simulink model "TRN_current"  (Simulink 6.2)
settings: Solver=ode45  SolverMode=SingleTasking  StartTime=0  StopTime=6  MaxStep=0.1  RelTol=1e-3  AbsTol=1e-3
libraries: simulink x1
(part 1 of 3)
settings Model: LastModifiedBy=mark
settings DataIOCC: LimitDataPoints=off  SaveOutput=off  SaveTime=off  Refine=5
settings OptimizationCC: BooleanDataType=off
settings HardwareCC: TargetUnknown=on
settings RTWCC: TemplateMakefile=grt_unix.tmf
settings GRTTargetCC: ModelReferenceCompliant=off  MatFileLogging=off

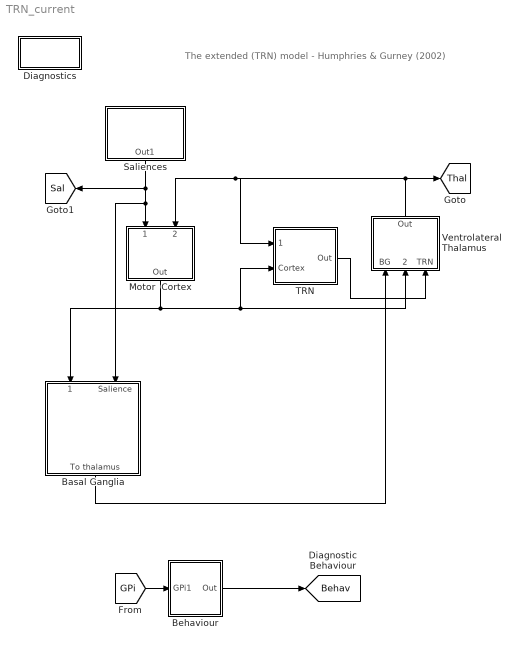
== system TRN_current ==
  note: The extended (TRN) model - Humphries & Gurney (2002)
  Basal Ganglia : Subsystem  Orientation=down  mask(Basal Ganglia){D2=0.2, D1=0.2}
      mask prompts: D2 "D2 base level"; D1 "D1 base level"
  Behaviour : Subsystem  mask(Behaviour expression){on_thresh=0.025, off_thresh=0.1}
      mask prompts: on_thresh "GPi level for behav. on"; off_thresh "GPi level for behav.  off"
  Diagnostics : Subsystem
  Motor  Cortex : Subsystem  Orientation=down  mask(Cortex){W_Thal=1, W_Sal=1, A_rate=25, slope=1, thresh=0}
      mask prompts: W_Thal "Thalamus input weight"; W_Sal "Salience input weight"; A_rate "membrane decay rate"; slope "output slope"; thresh "output thresh"
      mask help: 3 channel striatum - non-recurrent
  Saliences : Subsystem  Orientation=down
  TRN : Subsystem  mask(Thalamic Reticular Nucleus){W_Ctx=1, W_Thal=1, A_rate=25, slope=1, thresh=0}
      mask prompts: W_Ctx "Cortex input weight"; W_Thal "Thalamus input weight"; A_rate "membrane decay rate"; slope "output slope"; thresh "output thresh"
      mask help: 3 channel striatum - non-recurrent
  Ventrolateral Thalamus : Subsystem  Orientation=up  mask(Thalamus){W_TRNwit=-0.1, W_TRNdif=-0.7, W_Ctx=1, W_BG=-1, A_rate=25, slope=1, thresh=0}
      mask prompts: W_TRNwit "Within input weight"; W_TRNdif "Diffuse input weight"; W_Ctx "Cortex input weight"; W_BG "BG input weight"; A_rate "membrane decay rate"; slope "output slope"; thresh "output thresh"
      mask help: 3 channel striatum - non-recurrent
  tag scope: Behav=global, Sal=global, Thal=global
  wires:
  Ventrolateral Thalamus/1(Out) -> [Thal], Motor  Cortex/2(Thalamus), TRN/1(Thalamus)
  [GPi] -> Behaviour/1(GPi1)
  Behaviour/1(Out) -> [Behav]
  Saliences/1(Out1) -> [Sal], Motor  Cortex/1(Salience), Basal Ganglia/2(Salience)
  Motor  Cortex/1(Out) -> Basal Ganglia/1(From cortex), TRN/2(Cortex), Ventrolateral Thalamus/2(Cortex)
  Basal Ganglia/1(To thalamus) -> Ventrolateral Thalamus/1(BG)
  TRN/1(Out) -> Ventrolateral Thalamus/3(TRN)

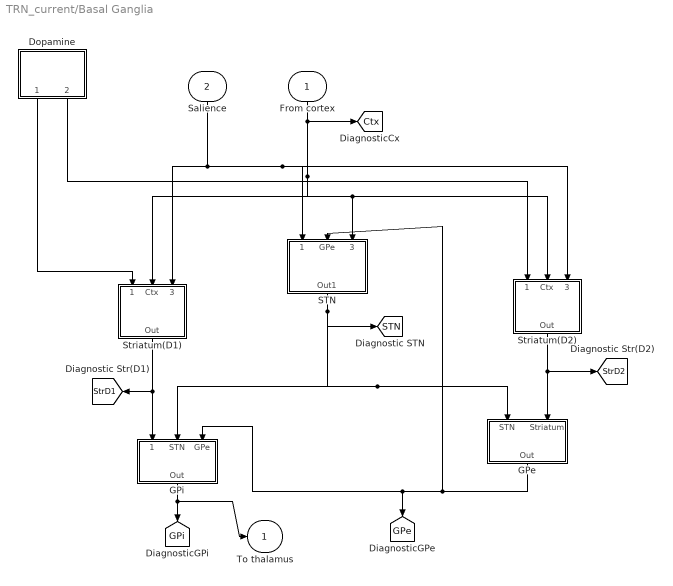
== system TRN_current/Basal Ganglia ==
  From cortex : Inport  Orientation=down  Port=1  SampleTime=0  LatchInput=off
  Salience : Inport  Orientation=down  Port=2  SampleTime=0  LatchInput=off
  Dopamine : Subsystem  Orientation=down
  GPe : Subsystem  Orientation=down  mask(GPe){W_str=-1, W_STN=0.8, A_rate=25, slope=1, thresh=-0.2}
      mask prompts: W_str "weight from Striatum"; W_STN "weight from STN (exc.)"; A_rate "membrane decay rate"; slope "output slope"; thresh "output thresh"
      mask help: 3 channel GPe
  GPi : Subsystem  Orientation=down  mask(GPi){W_str=-1, W_STN=0.8, W_GPe=-0.4, A_rate=25, slope=1, thresh=-0.2}
      mask prompts: W_str "weight from Str"; W_STN "weight from STN"; W_GPe "weight from GPe"; A_rate "membrane decay rate"; slope "output slope"; thresh "output thresh"
      mask help: 3 channel GPe
  STN : Subsystem  Orientation=down
  Striatum(D1) : Subsystem  Orientation=down  mask(Striatum (D1)){W_sal=0.5, W_ctx=0.5, A_rate=25, slope=1, thresh=0.2}
      mask prompts: W_sal "Salience input weight"; W_ctx "Cortex input weight"; A_rate "membrane decay rate"; slope "output slope"; thresh "output thresh"
      mask help: 3 channel striatum - non-recurrent
  Striatum(D2) : Subsystem  Orientation=down  mask(Striatum (D1)){W_sal=0.5, W_ctx=0.5, A_rate=25, slope=1, thresh=0.2}
      mask prompts: W_sal "Salience input weight"; W_ctx "Cortex input weight"; A_rate "membrane decay rate"; slope "output slope"; thresh "output thresh"
      mask help: 3 channel striatum - non-recurrent
  To thalamus : Outport
  tag scope: Ctx=global, GPe=global, GPi=global, STN=global, StrD1=global, StrD2=global
  wires:
  GPe/1(Out) -> STN/2(GPe), GPi/3(GPe), [GPe]
  Striatum(D2)/1(Out) -> GPe/2(Striatum), [StrD2]
  STN/1(Out1) -> [STN], GPe/1(STN), GPi/2(STN)
  Striatum(D1)/1(Out) -> GPi/1(Striatum), [StrD1]
  Dopamine/1(GPi(D1)) -> Striatum(D1)/1(Dopamine)
  Dopamine/2(GPe(D2)) -> Striatum(D2)/1(Dopamine)
  GPi/1(Out) -> [GPi], To thalamus/1
  Salience/1 -> Striatum(D1)/3(Salience), Striatum(D2)/3(Salience), STN/1(saliences)
  From cortex/1 -> [Ctx], Striatum(D1)/2(Ctx), Striatum(D2)/2(Ctx), STN/3(cortex)

== system TRN_current/Behaviour ==
  GPi1 : Inport  Port=1  LatchInput=off
  Constant : Constant
  Relay : Relay  OnSwitchValue=1 - on_thresh  OffSwitchValue=1 - off_thresh
  Sum : Sum  Inputs=+-  SaturateOnIntegerOverflow=on  InputSameDT=on
  Out : Outport  InitialOutput=0
  wires:
  Constant/1 -> Sum/1
  Sum/1 -> Relay/1
  GPi1/1 -> Sum/2
  Relay/1 -> Out/1

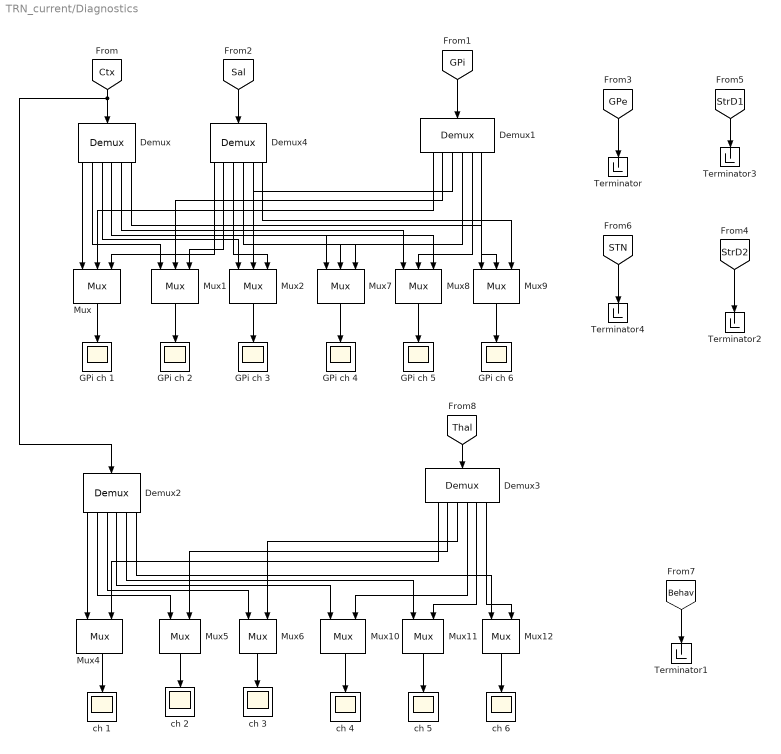
== system TRN_current/Diagnostics ==
  Demux{,1..4} (5 alike) : Demux  Orientation=down  Outputs=6
  GPi ch {1..6} (6 alike) : Scope
      GPi ch 1 settings: Orientation=down  TickLabels=on  YMin=0  YMax=1  SaveName=GPic1_6  DataFormat=Array  MaxDataPoints=7000
      GPi ch 2 settings: Orientation=down  TickLabels=on  YMin=0  YMax=1  SaveName=GPic2_6  DataFormat=Array  MaxDataPoints=7000
      GPi ch 3 settings: Orientation=down  TickLabels=on  YMin=0  YMax=1  SaveName=GPic3_6  DataFormat=Array
      GPi ch 4 settings: Orientation=down  TickLabels=on  YMin=0  YMax=0.75  SaveName=GPic4_6  DataFormat=Array
      GPi ch 5 settings: Orientation=down  TickLabels=on  YMin=0  YMax=0.75  SaveName=GPi3full  DataFormat=Array
      GPi ch 6 settings: Orientation=down  TickLabels=on  YMin=0  YMax=0.75  SaveName=GPi6full6  DataFormat=Array
  Mux{,1..2,7..9} (6 alike) : Mux  Orientation=down  Inputs=3
  Mux{4..6,10..12} (6 alike) : Mux  Orientation=down  Inputs=2
  Terminator{,1..4} (5 alike) : Terminator
      settings: Orientation=down
  ch {1..6} (6 alike) : Scope
      ch 1 settings: Orientation=down  TickLabels=on  YMin=0  YMax=1  SaveName=gpe1  DataFormat=Array
      ch 2 settings: Orientation=down  TickLabels=on  YMin=0  YMax=0.75  SaveName=gpe2  DataFormat=Array
      ch 3 settings: Orientation=down  TickLabels=on  YMin=0  YMax=0.75  SaveName=ch3  DataFormat=Array
      ch 4 settings: Orientation=down  TickLabels=on  YMin=0  YMax=0.75  SaveName=ch4  DataFormat=Array
      ch 5 settings: Orientation=down  TickLabels=on  YMin=0  YMax=0.75  SaveName=ch5  DataFormat=Array
      ch 6 settings: Orientation=down  TickLabels=on  YMin=0  YMax=0.75  SaveName=ch6  DataFormat=Array
  wires:
  [Thal] -> Demux3/1
  Mux/1 -> GPi ch 1/1
  Demux/1 -> Mux/1
  Demux/2 -> Mux1/1
  Mux1/1 -> GPi ch 2/1
  Mux2/1 -> GPi ch 3/1
  Demux/3 -> Mux2/1
  Demux/4 -> Mux7/1
  Demux/5 -> Mux8/1
  Demux/6 -> Mux9/1
  Demux1/3 -> Mux2/2
  [GPi] -> Demux1/1
  Demux1/1 -> Mux/2
  Demux1/2 -> Mux1/2
  Demux1/4 -> Mux7/2
  Demux1/5 -> Mux8/2
  Demux1/6 -> Mux9/2
  Mux7/1 -> GPi ch 4/1
  Mux8/1 -> GPi ch 5/1
  Mux9/1 -> GPi ch 6/1
  [Ctx] -> Demux/1, Demux2/1
  Mux4/1 -> ch 1/1
  Demux2/1 -> Mux4/1
  Demux2/2 -> Mux5/1
  Mux5/1 -> ch 2/1
  Mux6/1 -> ch 3/1
  Demux2/3 -> Mux6/1
  Demux2/4 -> Mux10/1
  Demux2/5 -> Mux11/1
  Demux2/6 -> Mux12/1
  Demux3/3 -> Mux6/2
  Demux3/1 -> Mux4/2
  Demux3/2 -> Mux5/2
  Demux3/4 -> Mux10/2
  Demux3/5 -> Mux11/2
  Demux3/6 -> Mux12/2
  Mux10/1 -> ch 4/1
  Mux11/1 -> ch 5/1
  Mux12/1 -> ch 6/1
  [Sal] -> Demux4/1
  Demux4/1 -> Mux/3
  Demux4/2 -> Mux1/3
  Demux4/3 -> Mux2/3
  Demux4/4 -> Mux7/3
  Demux4/5 -> Mux8/3
  Demux4/6 -> Mux9/3
  [GPe] -> Terminator/1
  [Behav] -> Terminator1/1
  [StrD2] -> Terminator2/1
  [StrD1] -> Terminator3/1
  [STN] -> Terminator4/1

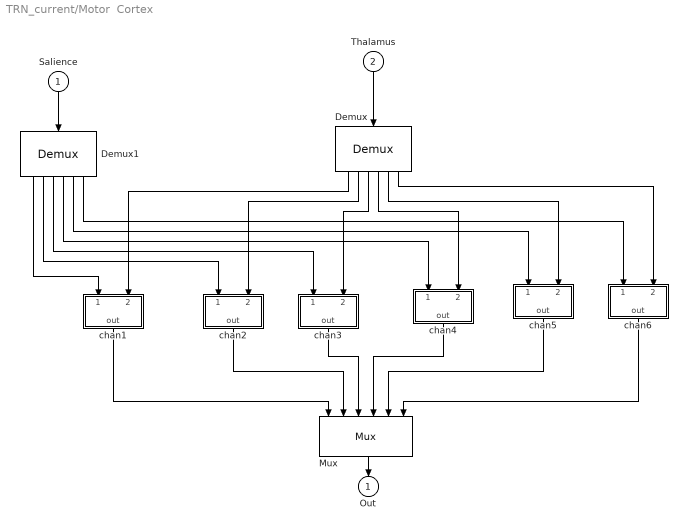
== system TRN_current/Motor  Cortex ==
  Salience : Inport  Orientation=down  Port=1  LatchInput=off
  Thalamus : Inport  Orientation=down  Port=2  LatchInput=off
  Demux : Demux  Orientation=down  Outputs=6
  Demux1 : Demux  Orientation=down  Outputs=6
  Mux : Mux  Orientation=down  Inputs=6
  chan1 : Subsystem  Orientation=down
  chan2 : Subsystem  Orientation=down
  chan3 : Subsystem  Orientation=down
  chan4 : Subsystem  Orientation=down
  chan5 : Subsystem  Orientation=down
  chan6 : Subsystem  Orientation=down
  Out : Outport  Orientation=down  InitialOutput=0
  wires:
  Demux1/1 -> chan1/1(Salience)
  Demux1/2 -> chan2/1(Salience)
  Demux1/3 -> chan3/1(Salience)
  Demux1/4 -> chan4/1(Salience)
  Demux1/5 -> chan5/1(Salience)
  Demux1/6 -> chan6/1(Salience)
  Salience/1 -> Demux1/1
  chan6/1(out) -> Mux/6
  chan5/1(out) -> Mux/5
  chan4/1(out) -> Mux/4
  Demux/6 -> chan6/2(Thalamus)
  Demux/5 -> chan5/2(Thalamus)
  Demux/4 -> chan4/2(Thalamus)
  Demux/3 -> chan3/2(Thalamus)
  Demux/2 -> chan2/2(Thalamus)
  Demux/1 -> chan1/2(Thalamus)
  chan2/1(out) -> Mux/2
  chan3/1(out) -> Mux/3
  Mux/1 -> Out/1
  Thalamus/1 -> Demux/1
  chan1/1(out) -> Mux/1

== system TRN_current/Saliences ==
  Do left : Constant  Orientation=down  Value=0
  Salience (simple) : Subsystem  Orientation=down
  Switch : Switch  Orientation=down  Threshold=0.5  SaturateOnIntegerOverflow=on  InputSameDT=on
  step pairs : Subsystem  Orientation=down
  Out1 : Outport  Orientation=down  InitialOutput=0
  wires:
  Switch/1 -> Out1/1
  Salience (simple)/1(out) -> Switch/3
  step pairs/1(out) -> Switch/1
  Do left/1 -> Switch/2

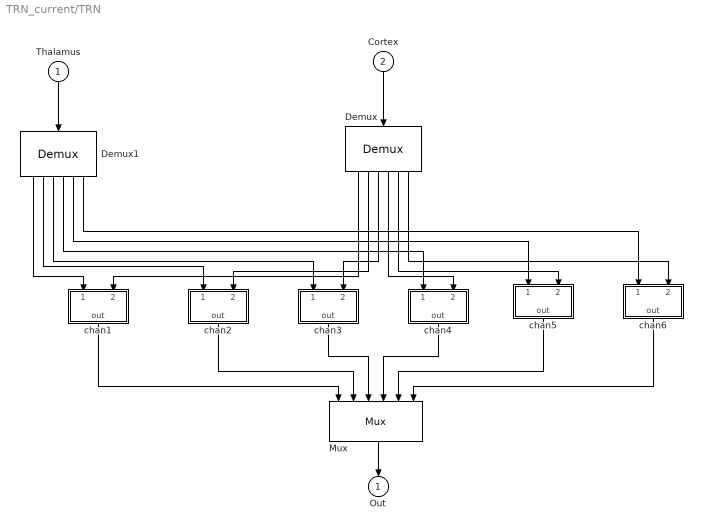
== system TRN_current/TRN ==
  Thalamus : Inport  Orientation=down  Port=1  LatchInput=off
  Cortex : Inport  Orientation=down  Port=2  LatchInput=off
  Demux : Demux  Orientation=down  Outputs=6
  Demux1 : Demux  Orientation=down  Outputs=6
  Mux : Mux  Orientation=down  Inputs=6
  chan1 : Subsystem  Orientation=down
  chan2 : Subsystem  Orientation=down
  chan3 : Subsystem  Orientation=down
  chan4 : Subsystem  Orientation=down
  chan5 : Subsystem  Orientation=down
  chan6 : Subsystem  Orientation=down
  Out : Outport  Orientation=down  InitialOutput=0
  wires:
  Demux/1 -> chan1/2(Cortex)
  Demux1/1 -> chan1/1(Thalamus)
  Mux/1 -> Out/1
  chan1/1(out) -> Mux/1
  chan3/1(out) -> Mux/3
  chan2/1(out) -> Mux/2
  chan4/1(out) -> Mux/4
  chan5/1(out) -> Mux/5
  chan6/1(out) -> Mux/6
  Cortex/1 -> Demux/1
  Thalamus/1 -> Demux1/1
  Demux1/2 -> chan2/1(Thalamus)
  Demux1/3 -> chan3/1(Thalamus)
  Demux1/4 -> chan4/1(Thalamus)
  Demux1/5 -> chan5/1(Thalamus)
  Demux1/6 -> chan6/1(Thalamus)
  Demux/2 -> chan2/2(Cortex)
  Demux/3 -> chan3/2(Cortex)
  Demux/4 -> chan4/2(Cortex)
  Demux/5 -> chan5/2(Cortex)
  Demux/6 -> chan6/2(Cortex)

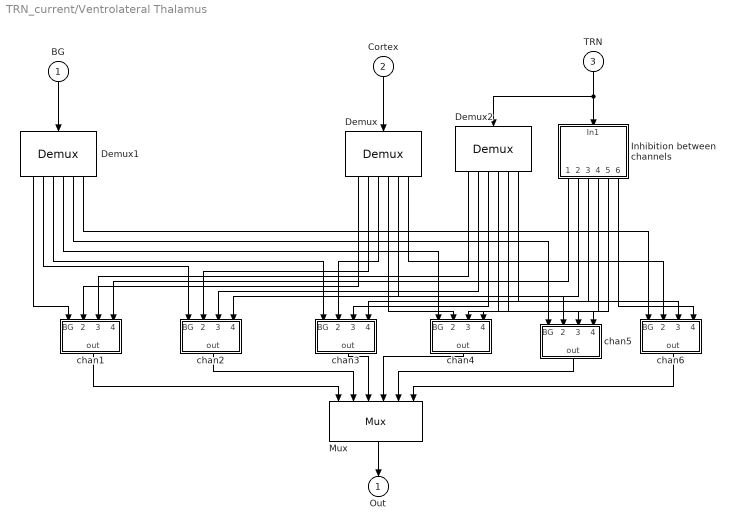
== system TRN_current/Ventrolateral Thalamus ==
  BG : Inport  Orientation=down  Port=1  LatchInput=off
  Cortex : Inport  Orientation=down  Port=2  LatchInput=off
  TRN : Inport  Orientation=down  Port=3  LatchInput=off
  Demux : Demux  Orientation=down  Outputs=6
  Demux1 : Demux  Orientation=down  Outputs=6
  Demux2 : Demux  Orientation=down  Outputs=6
  Inhibition between channels : Subsystem  Orientation=down
  Mux : Mux  Orientation=down  Inputs=6
  chan1 : Subsystem  Orientation=down
  chan2 : Subsystem  Orientation=down
  chan3 : Subsystem  Orientation=down
  chan4 : Subsystem  Orientation=down
  chan5 : Subsystem  Orientation=down
  chan6 : Subsystem  Orientation=down
  Out : Outport  Orientation=down  InitialOutput=0
  wires:
  Mux/1 -> Out/1
  chan1/1(out) -> Mux/1
  chan3/1(out) -> Mux/3
  chan2/1(out) -> Mux/2
  chan4/1(out) -> Mux/4
  chan5/1(out) -> Mux/5
  chan6/1(out) -> Mux/6
  BG/1 -> Demux1/1
  Demux1/2 -> chan2/1(BG)
  Demux1/3 -> chan3/1(BG)
  Demux1/4 -> chan4/1(BG)
  Demux1/5 -> chan5/1(BG)
  Cortex/1 -> Demux/1
  Demux1/6 -> chan6/1(BG)
  Demux1/1 -> chan1/1(BG)
  TRN/1 -> Inhibition between channels/1(In1), Demux2/1
  Demux2/1 -> chan1/3(TRN)
  Inhibition between channels/1(Out1) -> chan1/4(TRN1)
  Demux2/2 -> chan2/3(TRN)
  Demux2/3 -> chan3/3(TRN)
  Demux2/4 -> chan4/3(TRN)
  Demux2/5 -> chan5/3(TRN)
  Demux2/6 -> chan6/3(TRN)
  Inhibition between channels/2(Out2) -> chan2/4(TRN1)
  Inhibition between channels/3(Out3) -> chan3/4(TRN1)
  Inhibition between channels/4(Out4) -> chan4/4(TRN1)
  Inhibition between channels/5(Out5) -> chan5/4(TRN1)
  Inhibition between channels/6(Out6) -> chan6/4(TRN1)
  Demux/2 -> chan2/2(Cortex)
  Demux/3 -> chan3/2(Cortex)
  Demux/4 -> chan4/2(Cortex)
  Demux/5 -> chan5/2(Cortex)
  Demux/6 -> chan6/2(Cortex)
  Demux/1 -> chan1/2(Cortex)

== system TRN_current/Basal Ganglia/Dopamine ==
  D1 base level : Constant  Value=D1
  D2 base level : Constant  Orientation=left  Value=D2
  Mux : Mux  Orientation=down  Inputs=6
  Mux1 : Mux  Orientation=down  Inputs=6
  GPi(D1) : Outport  Orientation=down  InitialOutput=0
  GPe(D2) : Outport  Orientation=down  Port=2  InitialOutput=0
  wires:
  Mux1/1 -> GPe(D2)/1
  D2 base level/1 -> Mux1/6, Mux1/5, Mux1/4, Mux1/3, Mux1/2, Mux1/1
  Mux/1 -> GPi(D1)/1
  D1 base level/1 -> Mux/6, Mux/5, Mux/4, Mux/3, Mux/2, Mux/1

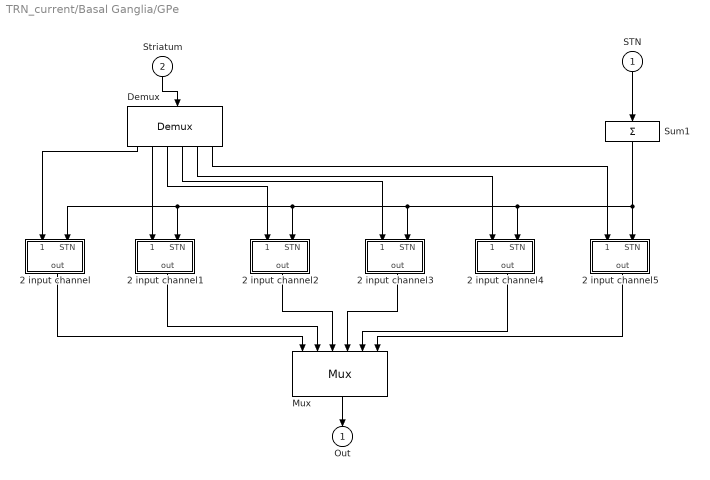
== system TRN_current/Basal Ganglia/GPe ==
  STN : Inport  Orientation=down  Port=1  LatchInput=off
  Striatum : Inport  Orientation=down  Port=2  LatchInput=off
  2 input channel : Subsystem  Orientation=down
  2 input channel1 : Subsystem  Orientation=down
  2 input channel2 : Subsystem  Orientation=down
  2 input channel3 : Subsystem  Orientation=down
  2 input channel4 : Subsystem  Orientation=down
  2 input channel5 : Subsystem  Orientation=down
  Demux : Demux  Orientation=down  Outputs=6
  Mux : Mux  Orientation=down  Inputs=6
  Sum1 : Sum  Orientation=down  Inputs=+  SaturateOnIntegerOverflow=on  InputSameDT=on
  Out : Outport  Orientation=down  InitialOutput=0
  wires:
  Sum1/1 -> 2 input channel5/2(STN), 2 input channel/2(STN), 2 input channel1/2(STN), 2 input channel2/2(STN), 2 input channel3/2(STN), 2 input channel4/2(STN)
  Demux/1 -> 2 input channel/1(Striatum)
  STN/1 -> Sum1/1
  2 input channel/1(out) -> Mux/1
  2 input channel1/1(out) -> Mux/2
  2 input channel2/1(out) -> Mux/3
  Mux/1 -> Out/1
  Striatum/1 -> Demux/1
  Demux/2 -> 2 input channel1/1(Striatum)
  Demux/3 -> 2 input channel2/1(Striatum)
  Demux/4 -> 2 input channel3/1(Striatum)
  Demux/5 -> 2 input channel4/1(Striatum)
  Demux/6 -> 2 input channel5/1(Striatum)
  2 input channel3/1(out) -> Mux/4
  2 input channel4/1(out) -> Mux/5
  2 input channel5/1(out) -> Mux/6

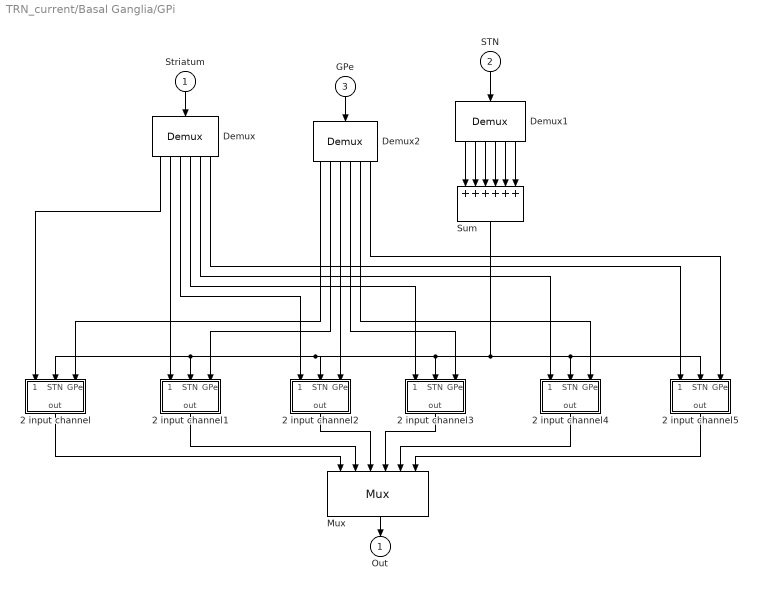
== system TRN_current/Basal Ganglia/GPi ==
  Striatum : Inport  Orientation=down  Port=1  LatchInput=off
  STN : Inport  Orientation=down  Port=2  LatchInput=off
  GPe : Inport  Orientation=down  Port=3  LatchInput=off
  2 input channel : Subsystem  Orientation=down
  2 input channel1 : Subsystem  Orientation=down
  2 input channel2 : Subsystem  Orientation=down
  2 input channel3 : Subsystem  Orientation=down
  2 input channel4 : Subsystem  Orientation=down
  2 input channel5 : Subsystem  Orientation=down
  Demux : Demux  Orientation=down  Outputs=6
  Demux1 : Demux  Orientation=down  Outputs=6
  Demux2 : Demux  Orientation=down  Outputs=6
  Mux : Mux  Orientation=down  Inputs=6
  Sum : Sum  Orientation=down  Inputs=++++++  SaturateOnIntegerOverflow=on  InputSameDT=on
  Out : Outport  Orientation=down  InitialOutput=0
  wires:
  Mux/1 -> Out/1
  2 input channel2/1(out) -> Mux/3
  2 input channel1/1(out) -> Mux/2
  2 input channel/1(out) -> Mux/1
  GPe/1 -> Demux2/1
  Demux2/1 -> 2 input channel/3(GPe)
  Demux2/2 -> 2 input channel1/3(GPe)
  Demux2/3 -> 2 input channel2/3(GPe)
  Demux/2 -> 2 input channel1/1(Striatum)
  Demux/1 -> 2 input channel/1(Striatum)
  Striatum/1 -> Demux/1
  Demux/3 -> 2 input channel2/1(Striatum)
  Demux/4 -> 2 input channel3/1(Striatum)
  Demux/5 -> 2 input channel4/1(Striatum)
  Demux/6 -> 2 input channel5/1(Striatum)
  Demux2/4 -> 2 input channel3/3(GPe)
  Demux2/5 -> 2 input channel4/3(GPe)
  Demux1/1 -> Sum/1
  Demux1/2 -> Sum/2
  Demux1/3 -> Sum/3
  Demux1/4 -> Sum/4
  Demux1/5 -> Sum/5
  Demux1/6 -> Sum/6
  STN/1 -> Demux1/1
  Sum/1 -> 2 input channel/2(STN), 2 input channel1/2(STN), 2 input channel2/2(STN), 2 input channel3/2(STN), 2 input channel4/2(STN), 2 input channel5/2(STN)
  Demux2/6 -> 2 input channel5/3(GPe)
  2 input channel3/1(out) -> Mux/4
  2 input channel4/1(out) -> Mux/5
  2 input channel5/1(out) -> Mux/6

== system TRN_current/Basal Ganglia/STN ==
  saliences : Inport  Orientation=down  Port=1  LatchInput=off
  GPe : Inport  Orientation=down  Port=2  LatchInput=off
  cortex : Inport  Orientation=down  Port=3  LatchInput=off
  STN discrete model : Subsystem  Orientation=down  mask(STN){W_sal=0.5, W_Ctx=0.5, W_GPe=-1, A_rate=25, slope=1, thresh=-0.25}
      mask prompts: W_sal "weight from salience"; W_Ctx "weight from Cortex"; W_GPe "weight from GPe(inhib.)"; A_rate "membrane decay rate"; slope "output slope"; thresh "output thresh"
      mask help: 3 channel GPe
  Out1 : Outport  Orientation=down  InitialOutput=0
  wires:
  GPe/1 -> STN discrete model/2(GPe)
  saliences/1 -> STN discrete model/1(Saliences)
  STN discrete model/1(Out) -> Out1/1
  cortex/1 -> STN discrete model/3(Cortex)

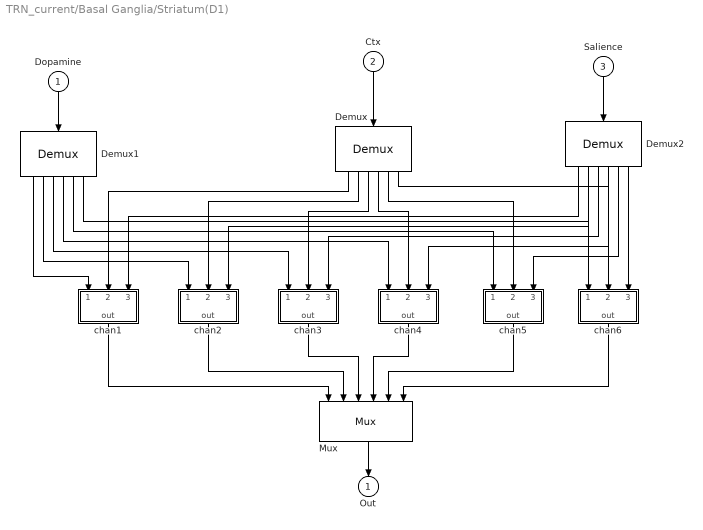
== system TRN_current/Basal Ganglia/Striatum(D1) ==
  Dopamine : Inport  Orientation=down  Port=1  LatchInput=off
  Ctx : Inport  Orientation=down  Port=2  LatchInput=off
  Salience : Inport  Orientation=down  Port=3  LatchInput=off
  Demux : Demux  Orientation=down  Outputs=6
  Demux1 : Demux  Orientation=down  Outputs=6
  Demux2 : Demux  Orientation=down  Outputs=6
  Mux : Mux  Orientation=down  Inputs=6
  chan1 : Subsystem  Orientation=down
  chan2 : Subsystem  Orientation=down
  chan3 : Subsystem  Orientation=down
  chan4 : Subsystem  Orientation=down
  chan5 : Subsystem  Orientation=down
  chan6 : Subsystem  Orientation=down
  Out : Outport  Orientation=down  InitialOutput=0
  wires:
  Ctx/1 -> Demux/1
  Mux/1 -> Out/1
  chan1/1(out) -> Mux/1
  chan3/1(out) -> Mux/3
  chan2/1(out) -> Mux/2
  Demux/2 -> chan2/2(cortex)
  Demux/3 -> chan3/2(cortex)
  Demux/4 -> chan4/2(cortex)
  Demux/5 -> chan5/2(cortex)
  Demux/6 -> chan6/2(cortex)
  chan4/1(out) -> Mux/4
  chan5/1(out) -> Mux/5
  chan6/1(out) -> Mux/6
  Dopamine/1 -> Demux1/1
  Demux1/6 -> chan6/1(dopamine)
  Demux1/5 -> chan5/1(dopamine)
  Demux1/4 -> chan4/1(dopamine)
  Demux1/3 -> chan3/1(dopamine)
  Demux1/2 -> chan2/1(dopamine)
  Demux1/1 -> chan1/1(dopamine)
  Salience/1 -> Demux2/1
  Demux2/2 -> chan2/3(salience)
  Demux2/3 -> chan3/3(salience)
  Demux2/4 -> chan4/3(salience)
  Demux2/5 -> chan5/3(salience)
  Demux2/6 -> chan6/3(salience)
  Demux/1 -> chan1/2(cortex)
  Demux2/1 -> chan1/3(salience)

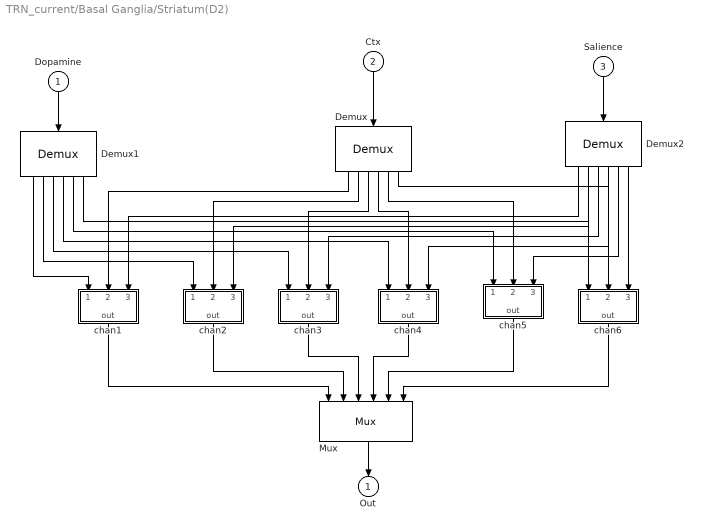
== system TRN_current/Basal Ganglia/Striatum(D2) ==
  Dopamine : Inport  Orientation=down  Port=1  LatchInput=off
  Ctx : Inport  Orientation=down  Port=2  LatchInput=off
  Salience : Inport  Orientation=down  Port=3  LatchInput=off
  Demux : Demux  Orientation=down  Outputs=6
  Demux1 : Demux  Orientation=down  Outputs=6
  Demux2 : Demux  Orientation=down  Outputs=6
  Mux : Mux  Orientation=down  Inputs=6
  chan1 : Subsystem  Orientation=down
  chan2 : Subsystem  Orientation=down
  chan3 : Subsystem  Orientation=down
  chan4 : Subsystem  Orientation=down
  chan5 : Subsystem  Orientation=down
  chan6 : Subsystem  Orientation=down
  Out : Outport  Orientation=down  InitialOutput=0
  wires:
  Demux2/1 -> chan1/3(salience)
  Demux/1 -> chan1/2(cortex)
  Demux2/6 -> chan6/3(salience)
  Demux2/5 -> chan5/3(salience)
  Demux2/4 -> chan4/3(salience)
  Demux2/3 -> chan3/3(salience)
  Demux2/2 -> chan2/3(salience)
  Salience/1 -> Demux2/1
  Demux1/1 -> chan1/1(dopamine)
  Demux1/2 -> chan2/1(dopamine)
  Demux1/3 -> chan3/1(dopamine)
  Demux1/4 -> chan4/1(dopamine)
  Demux1/5 -> chan5/1(dopamine)
  Demux1/6 -> chan6/1(dopamine)
  Dopamine/1 -> Demux1/1
  chan6/1(out) -> Mux/6
  chan5/1(out) -> Mux/5
  chan4/1(out) -> Mux/4
  Demux/6 -> chan6/2(cortex)
  Demux/5 -> chan5/2(cortex)
  Demux/4 -> chan4/2(cortex)
  Demux/3 -> chan3/2(cortex)
  Demux/2 -> chan2/2(cortex)
  chan2/1(out) -> Mux/2
  chan3/1(out) -> Mux/3
  chan1/1(out) -> Mux/1
  Mux/1 -> Out/1
  Ctx/1 -> Demux/1

== system TRN_current/Motor  Cortex/chan1 ==
  Salience : Inport  Orientation=down  Port=1  PortDimensions=1  LatchInput=off
  Thalamus : Inport  Orientation=down  Port=2  LatchInput=off
  Sum : Sum  Orientation=down  SaturateOnIntegerOverflow=on  InputSameDT=on
  leaky integration : Subsystem  Orientation=down
  piecewise lin.1 : S-Function  Orientation=down  FunctionName=Mpieclin  Parameters=slope,thresh
  weight : Gain  Orientation=down  Gain=W_Thal  SaturateOnIntegerOverflow=on
  weight1 : Gain  Orientation=down  Gain=W_Sal  SaturateOnIntegerOverflow=on
  out : Outport  Orientation=down  InitialOutput=0
  wires:
  Thalamus/1 -> weight/1
  Salience/1 -> weight1/1
  weight/1 -> Sum/2
  weight1/1 -> Sum/1
  piecewise lin.1/1 -> out/1
  Sum/1 -> leaky integration/1(Inport)
  leaky integration/1(Outport) -> piecewise lin.1/1

== system TRN_current/Motor  Cortex/chan2 ==
  Salience : Inport  Orientation=down  Port=1  PortDimensions=1  LatchInput=off
  Thalamus : Inport  Orientation=down  Port=2  LatchInput=off
  Sum : Sum  Orientation=down  SaturateOnIntegerOverflow=on  InputSameDT=on
  leaky integration : Subsystem  Orientation=down
  piecewise lin.1 : S-Function  Orientation=down  FunctionName=Mpieclin  Parameters=slope,thresh
  weight : Gain  Orientation=down  Gain=W_Thal  SaturateOnIntegerOverflow=on
  weight1 : Gain  Orientation=down  Gain=W_Sal  SaturateOnIntegerOverflow=on
  out : Outport  Orientation=down  InitialOutput=0
  wires:
  leaky integration/1(Outport) -> piecewise lin.1/1
  Sum/1 -> leaky integration/1(Inport)
  piecewise lin.1/1 -> out/1
  weight1/1 -> Sum/1
  weight/1 -> Sum/2
  Salience/1 -> weight1/1
  Thalamus/1 -> weight/1

== system TRN_current/Motor  Cortex/chan3 ==
  Salience : Inport  Orientation=down  Port=1  PortDimensions=1  LatchInput=off
  Thalamus : Inport  Orientation=down  Port=2  LatchInput=off
  Sum : Sum  Orientation=down  SaturateOnIntegerOverflow=on  InputSameDT=on
  leaky integration : Subsystem  Orientation=down
  piecewise lin.1 : S-Function  Orientation=down  FunctionName=Mpieclin  Parameters=slope,thresh
  weight : Gain  Orientation=down  Gain=W_Thal  SaturateOnIntegerOverflow=on
  weight1 : Gain  Orientation=down  Gain=W_Sal  SaturateOnIntegerOverflow=on
  out : Outport  Orientation=down  InitialOutput=0
  wires:
  Thalamus/1 -> weight/1
  Salience/1 -> weight1/1
  weight/1 -> Sum/2
  weight1/1 -> Sum/1
  piecewise lin.1/1 -> out/1
  Sum/1 -> leaky integration/1(Inport)
  leaky integration/1(Outport) -> piecewise lin.1/1

== system TRN_current/Motor  Cortex/chan4 ==
  Salience : Inport  Orientation=down  Port=1  PortDimensions=1  LatchInput=off
  Thalamus : Inport  Orientation=down  Port=2  LatchInput=off
  Sum : Sum  Orientation=down  SaturateOnIntegerOverflow=on  InputSameDT=on
  leaky integration : Subsystem  Orientation=down
  piecewise lin.1 : S-Function  Orientation=down  FunctionName=Mpieclin  Parameters=slope,thresh
  weight : Gain  Orientation=down  Gain=W_Thal  SaturateOnIntegerOverflow=on
  weight1 : Gain  Orientation=down  Gain=W_Sal  SaturateOnIntegerOverflow=on
  out : Outport  Orientation=down  InitialOutput=0
  wires:
  leaky integration/1(Outport) -> piecewise lin.1/1
  Sum/1 -> leaky integration/1(Inport)
  piecewise lin.1/1 -> out/1
  weight1/1 -> Sum/1
  weight/1 -> Sum/2
  Salience/1 -> weight1/1
  Thalamus/1 -> weight/1

== system TRN_current/Motor  Cortex/chan5 ==
  Salience : Inport  Orientation=down  Port=1  PortDimensions=1  LatchInput=off
  Thalamus : Inport  Orientation=down  Port=2  LatchInput=off
  Sum : Sum  Orientation=down  SaturateOnIntegerOverflow=on  InputSameDT=on
  leaky integration : Subsystem  Orientation=down
  piecewise lin.1 : S-Function  Orientation=down  FunctionName=Mpieclin  Parameters=slope,thresh
  weight : Gain  Orientation=down  Gain=W_Thal  SaturateOnIntegerOverflow=on
  weight1 : Gain  Orientation=down  Gain=W_Sal  SaturateOnIntegerOverflow=on
  out : Outport  Orientation=down  InitialOutput=0
  wires:
  Thalamus/1 -> weight/1
  Salience/1 -> weight1/1
  weight/1 -> Sum/2
  weight1/1 -> Sum/1
  piecewise lin.1/1 -> out/1
  Sum/1 -> leaky integration/1(Inport)
  leaky integration/1(Outport) -> piecewise lin.1/1

== system TRN_current/Motor  Cortex/chan6 ==
  Salience : Inport  Orientation=down  Port=1  PortDimensions=1  LatchInput=off
  Thalamus : Inport  Orientation=down  Port=2  LatchInput=off
  Sum : Sum  Orientation=down  SaturateOnIntegerOverflow=on  InputSameDT=on
  leaky integration : Subsystem  Orientation=down
  piecewise lin.1 : S-Function  Orientation=down  FunctionName=Mpieclin  Parameters=slope,thresh
  weight : Gain  Orientation=down  Gain=W_Thal  SaturateOnIntegerOverflow=on
  weight1 : Gain  Orientation=down  Gain=W_Sal  SaturateOnIntegerOverflow=on
  out : Outport  Orientation=down  InitialOutput=0
  wires:
  leaky integration/1(Outport) -> piecewise lin.1/1
  Sum/1 -> leaky integration/1(Inport)
  piecewise lin.1/1 -> out/1
  weight1/1 -> Sum/1
  weight/1 -> Sum/2
  Salience/1 -> weight1/1
  Thalamus/1 -> weight/1

== system TRN_current/Saliences/Salience (simple) ==
  Saliences : DiscretePulseGenerator  Orientation=down  PulseType=Time based  Amplitude=[0.4 0.42 0.0 0.0 0.0 0.0]  Period=10  PulseWidth=[90 90 90 90 90 90]  PhaseDelay=[1 1 4 3 3 4]
  Sum : Sum  Orientation=down  SaturateOnIntegerOverflow=on  InputSameDT=on
  Transients : DiscretePulseGenerator  Orientation=down  PulseType=Time based  Amplitude=[0.2 0.0 0 0 0 0]  Period=10  PulseWidth=[10 30 10 10 10 10]  PhaseDelay=[4 5 10 10 10 10]
  out : Outport  Orientation=down  InitialOutput=0
  wires:
  ? -> Sum/2
  Sum/1 -> out/1
  Saliences/1 -> Sum/1

== system TRN_current/Saliences/step pairs ==
  Constant : Constant  Orientation=down  Value=[0 0 0 0 ]
  Constant1 : Constant  Orientation=down  Value=0.4
  Mux : Mux  Orientation=down  Inputs=3
  Repeating Sequence : simulink/Sources/Repeating Sequence  Orientation=down  rep_seq_t=[0 0.5 1.0 1.5 2.0 2.5 3.0 3.5 4 4.5 5]  rep_seq_y=[0 0.1 0.2 0.3 0.4 0.5 0.6 0.7 0.8 0.9 1]
  Scope : Scope
      settings: TickLabels=on  DataFormat=Array
  Zero-Order Hold : ZeroOrderHold  Orientation=down  SampleTime=0.5
  out : Outport  Orientation=down  InitialOutput=0
  wires:
  Mux/1 -> out/1, Scope/1
  Constant/1 -> Mux/3
  Repeating Sequence/1 -> Zero-Order Hold/1
  Zero-Order Hold/1 -> Mux/2
  Constant1/1 -> Mux/1

== system TRN_current/TRN/chan1 ==
  Thalamus : Inport  Orientation=down  Port=1  LatchInput=off
  Cortex : Inport  Orientation=down  Port=2  LatchInput=off
  Sum : Sum  Orientation=down  SaturateOnIntegerOverflow=on  InputSameDT=on
  leaky integration : Subsystem  Orientation=down
  piecewise lin. : S-Function  Orientation=down  FunctionName=Mpieclin  Parameters=slope,thresh
  weight : Gain  Orientation=down  Gain=W_Ctx  SaturateOnIntegerOverflow=on
  weight1 : Gain  Orientation=down  Gain=W_Thal  SaturateOnIntegerOverflow=on
  out : Outport  Orientation=down  InitialOutput=0
  wires:
  Cortex/1 -> weight/1
  leaky integration/1(Outport) -> piecewise lin./1
  weight1/1 -> Sum/1
  weight/1 -> Sum/2
  Sum/1 -> leaky integration/1(Inport)
  piecewise lin./1 -> out/1
  Thalamus/1 -> weight1/1

== system TRN_current/TRN/chan2 ==
  Thalamus : Inport  Orientation=down  Port=1  LatchInput=off
  Cortex : Inport  Orientation=down  Port=2  LatchInput=off
  Sum : Sum  Orientation=down  SaturateOnIntegerOverflow=on  InputSameDT=on
  leaky integration : Subsystem  Orientation=down
  piecewise lin. : S-Function  Orientation=down  FunctionName=Mpieclin  Parameters=slope,thresh
  weight : Gain  Orientation=down  Gain=W_Ctx  SaturateOnIntegerOverflow=on
  weight1 : Gain  Orientation=down  Gain=W_Thal  SaturateOnIntegerOverflow=on
  out : Outport  Orientation=down  InitialOutput=0
  wires:
  Thalamus/1 -> weight1/1
  piecewise lin./1 -> out/1
  Sum/1 -> leaky integration/1(Inport)
  weight/1 -> Sum/2
  weight1/1 -> Sum/1
  leaky integration/1(Outport) -> piecewise lin./1
  Cortex/1 -> weight/1

== system TRN_current/TRN/chan3 ==
  Thalamus : Inport  Orientation=down  Port=1  LatchInput=off
  Cortex : Inport  Orientation=down  Port=2  LatchInput=off
  Sum : Sum  Orientation=down  SaturateOnIntegerOverflow=on  InputSameDT=on
  leaky integration : Subsystem  Orientation=down
  piecewise lin. : S-Function  Orientation=down  FunctionName=Mpieclin  Parameters=slope,thresh
  weight : Gain  Orientation=down  Gain=W_Ctx  SaturateOnIntegerOverflow=on
  weight1 : Gain  Orientation=down  Gain=W_Thal  SaturateOnIntegerOverflow=on
  out : Outport  Orientation=down  InitialOutput=0
  wires:
  Cortex/1 -> weight/1
  leaky integration/1(Outport) -> piecewise lin./1
  weight1/1 -> Sum/1
  weight/1 -> Sum/2
  Sum/1 -> leaky integration/1(Inport)
  piecewise lin./1 -> out/1
  Thalamus/1 -> weight1/1

== system TRN_current/TRN/chan4 ==
  Thalamus : Inport  Orientation=down  Port=1  LatchInput=off
  Cortex : Inport  Orientation=down  Port=2  LatchInput=off
  Sum : Sum  Orientation=down  SaturateOnIntegerOverflow=on  InputSameDT=on
  leaky integration : Subsystem  Orientation=down
  piecewise lin. : S-Function  Orientation=down  FunctionName=Mpieclin  Parameters=slope,thresh
  weight : Gain  Orientation=down  Gain=W_Ctx  SaturateOnIntegerOverflow=on
  weight1 : Gain  Orientation=down  Gain=W_Thal  SaturateOnIntegerOverflow=on
  out : Outport  Orientation=down  InitialOutput=0
  wires:
  Thalamus/1 -> weight1/1
  piecewise lin./1 -> out/1
  Sum/1 -> leaky integration/1(Inport)
  weight/1 -> Sum/2
  weight1/1 -> Sum/1
  leaky integration/1(Outport) -> piecewise lin./1
  Cortex/1 -> weight/1

== system TRN_current/TRN/chan5 ==
  Thalamus : Inport  Orientation=down  Port=1  LatchInput=off
  Cortex : Inport  Orientation=down  Port=2  LatchInput=off
  Sum : Sum  Orientation=down  SaturateOnIntegerOverflow=on  InputSameDT=on
  leaky integration : Subsystem  Orientation=down
  piecewise lin. : S-Function  Orientation=down  FunctionName=Mpieclin  Parameters=slope,thresh
  weight : Gain  Orientation=down  Gain=W_Ctx  SaturateOnIntegerOverflow=on
  weight1 : Gain  Orientation=down  Gain=W_Thal  SaturateOnIntegerOverflow=on
  out : Outport  Orientation=down  InitialOutput=0
  wires:
  Cortex/1 -> weight/1
  leaky integration/1(Outport) -> piecewise lin./1
  weight1/1 -> Sum/1
  weight/1 -> Sum/2
  Sum/1 -> leaky integration/1(Inport)
  piecewise lin./1 -> out/1
  Thalamus/1 -> weight1/1

== system TRN_current/TRN/chan6 ==
  Thalamus : Inport  Orientation=down  Port=1  LatchInput=off
  Cortex : Inport  Orientation=down  Port=2  LatchInput=off
  Sum : Sum  Orientation=down  SaturateOnIntegerOverflow=on  InputSameDT=on
  leaky integration : Subsystem  Orientation=down
  piecewise lin. : S-Function  Orientation=down  FunctionName=Mpieclin  Parameters=slope,thresh
  weight : Gain  Orientation=down  Gain=W_Ctx  SaturateOnIntegerOverflow=on
  weight1 : Gain  Orientation=down  Gain=W_Thal  SaturateOnIntegerOverflow=on
  out : Outport  Orientation=down  InitialOutput=0
  wires:
  Thalamus/1 -> weight1/1
  piecewise lin./1 -> out/1
  Sum/1 -> leaky integration/1(Inport)
  weight/1 -> Sum/2
  weight1/1 -> Sum/1
  leaky integration/1(Outport) -> piecewise lin./1
  Cortex/1 -> weight/1

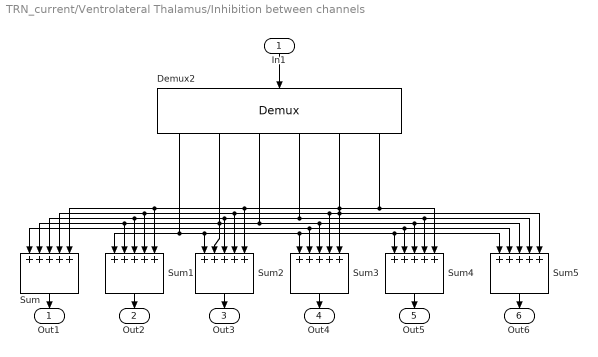
== system TRN_current/Ventrolateral Thalamus/Inhibition between channels ==
  In1 : Inport  Orientation=down  Port=1  LatchInput=off
  Demux2 : Demux  Orientation=down  Outputs=6
  Sum{,1..5} (6 alike) : Sum  Orientation=down  Inputs=+++++  SaturateOnIntegerOverflow=on  InputSameDT=on
  Out1 : Outport  Orientation=down  InitialOutput=0
  Out2 : Outport  Orientation=down  Port=2  InitialOutput=0
  Out3 : Outport  Orientation=down  Port=3  InitialOutput=0
  Out4 : Outport  Orientation=down  Port=4  InitialOutput=0
  Out5 : Outport  Orientation=down  Port=5  InitialOutput=0
  Out6 : Outport  Orientation=down  Port=6  InitialOutput=0
  wires:
  In1/1 -> Demux2/1
  Sum/1 -> Out1/1
  Demux2/2 -> Sum/1, Sum2/2, Sum3/2, Sum4/2, Sum5/2
  Demux2/1 -> Sum1/1, Sum2/1, Sum3/1, Sum4/1, Sum5/1
  Demux2/3 -> Sum/2, Sum1/2, Sum3/3, Sum4/3, Sum5/3
  Demux2/4 -> Sum/3, Sum1/3, Sum2/3, Sum4/4, Sum5/4
  Demux2/5 -> Sum/4, Sum1/4, Sum2/4, Sum3/4, Sum5/5
  Demux2/6 -> Sum/5, Sum1/5, Sum2/5, Sum3/5, Sum4/5
  Sum1/1 -> Out2/1
  Sum2/1 -> Out3/1
  Sum3/1 -> Out4/1
  Sum4/1 -> Out5/1
  Sum5/1 -> Out6/1

== system TRN_current/Ventrolateral Thalamus/chan1 ==
  BG : Inport  Orientation=down  Port=1  LatchInput=off
  Cortex : Inport  Orientation=down  Port=2  LatchInput=off
  TRN : Inport  Orientation=down  Port=3  LatchInput=off
  TRN1 : Inport  Orientation=down  Port=4  LatchInput=off
  Sum : Sum  Orientation=down  Inputs=++++  SaturateOnIntegerOverflow=on  InputSameDT=on
  leaky integration : Subsystem  Orientation=down
  piecewise lin. : S-Function  Orientation=down  FunctionName=Mpieclin  Parameters=slope,thresh
  weight : Gain  Orientation=down  Gain=W_Ctx  SaturateOnIntegerOverflow=on
  weight1 : Gain  Orientation=down  Gain=W_BG  SaturateOnIntegerOverflow=on
  weight2 : Gain  Orientation=down  Gain=W_TRNwit  SaturateOnIntegerOverflow=on
  weight3 : Gain  Orientation=down  Gain=W_TRNdif  SaturateOnIntegerOverflow=on
  out : Outport  Orientation=down  InitialOutput=0
  wires:
  leaky integration/1(Outport) -> piecewise lin./1
  weight1/1 -> Sum/1
  weight/1 -> Sum/2
  BG/1 -> weight1/1
  Cortex/1 -> weight/1
  weight2/1 -> Sum/3
  TRN/1 -> weight2/1
  TRN1/1 -> weight3/1
  weight3/1 -> Sum/4
  Sum/1 -> leaky integration/1(Inport)
  piecewise lin./1 -> out/1

== system TRN_current/Ventrolateral Thalamus/chan2 ==
  BG : Inport  Orientation=down  Port=1  LatchInput=off
  Cortex : Inport  Orientation=down  Port=2  LatchInput=off
  TRN : Inport  Orientation=down  Port=3  LatchInput=off
  TRN1 : Inport  Orientation=down  Port=4  LatchInput=off
  Sum : Sum  Orientation=down  Inputs=++++  SaturateOnIntegerOverflow=on  InputSameDT=on
  leaky integration : Subsystem  Orientation=down
  piecewise lin. : S-Function  Orientation=down  FunctionName=Mpieclin  Parameters=slope,thresh
  weight : Gain  Orientation=down  Gain=W_Ctx  SaturateOnIntegerOverflow=on
  weight1 : Gain  Orientation=down  Gain=W_BG  SaturateOnIntegerOverflow=on
  weight2 : Gain  Orientation=down  Gain=W_TRNwit  SaturateOnIntegerOverflow=on
  weight3 : Gain  Orientation=down  Gain=W_TRNdif  SaturateOnIntegerOverflow=on
  out : Outport  Orientation=down  InitialOutput=0
  wires:
  piecewise lin./1 -> out/1
  Sum/1 -> leaky integration/1(Inport)
  weight3/1 -> Sum/4
  TRN1/1 -> weight3/1
  TRN/1 -> weight2/1
  weight2/1 -> Sum/3
  Cortex/1 -> weight/1
  BG/1 -> weight1/1
  weight/1 -> Sum/2
  weight1/1 -> Sum/1
  leaky integration/1(Outport) -> piecewise lin./1

== system TRN_current/Ventrolateral Thalamus/chan3 ==
  BG : Inport  Orientation=down  Port=1  LatchInput=off
  Cortex : Inport  Orientation=down  Port=2  LatchInput=off
  TRN : Inport  Orientation=down  Port=3  LatchInput=off
  TRN1 : Inport  Orientation=down  Port=4  LatchInput=off
  Sum : Sum  Orientation=down  Inputs=++++  SaturateOnIntegerOverflow=on  InputSameDT=on
  leaky integration : Subsystem  Orientation=down
  piecewise lin. : S-Function  Orientation=down  FunctionName=Mpieclin  Parameters=slope,thresh
  weight : Gain  Orientation=down  Gain=W_Ctx  SaturateOnIntegerOverflow=on
  weight1 : Gain  Orientation=down  Gain=W_BG  SaturateOnIntegerOverflow=on
  weight2 : Gain  Orientation=down  Gain=W_TRNwit  SaturateOnIntegerOverflow=on
  weight3 : Gain  Orientation=down  Gain=W_TRNdif  SaturateOnIntegerOverflow=on
  out : Outport  Orientation=down  InitialOutput=0
  wires:
  leaky integration/1(Outport) -> piecewise lin./1
  weight1/1 -> Sum/1
  weight/1 -> Sum/2
  BG/1 -> weight1/1
  Cortex/1 -> weight/1
  weight2/1 -> Sum/3
  TRN/1 -> weight2/1
  TRN1/1 -> weight3/1
  weight3/1 -> Sum/4
  Sum/1 -> leaky integration/1(Inport)
  piecewise lin./1 -> out/1

== system TRN_current/Ventrolateral Thalamus/chan4 ==
  BG : Inport  Orientation=down  Port=1  LatchInput=off
  Cortex : Inport  Orientation=down  Port=2  LatchInput=off
  TRN : Inport  Orientation=down  Port=3  LatchInput=off
  TRN1 : Inport  Orientation=down  Port=4  LatchInput=off
  Sum : Sum  Orientation=down  Inputs=++++  SaturateOnIntegerOverflow=on  InputSameDT=on
  leaky integration : Subsystem  Orientation=down
  piecewise lin. : S-Function  Orientation=down  FunctionName=Mpieclin  Parameters=slope,thresh
  weight : Gain  Orientation=down  Gain=W_Ctx  SaturateOnIntegerOverflow=on
  weight1 : Gain  Orientation=down  Gain=W_BG  SaturateOnIntegerOverflow=on
  weight2 : Gain  Orientation=down  Gain=W_TRNwit  SaturateOnIntegerOverflow=on
  weight3 : Gain  Orientation=down  Gain=W_TRNdif  SaturateOnIntegerOverflow=on
  out : Outport  Orientation=down  InitialOutput=0
  wires:
  piecewise lin./1 -> out/1
  Sum/1 -> leaky integration/1(Inport)
  weight3/1 -> Sum/4
  TRN1/1 -> weight3/1
  TRN/1 -> weight2/1
  weight2/1 -> Sum/3
  Cortex/1 -> weight/1
  BG/1 -> weight1/1
  weight/1 -> Sum/2
  weight1/1 -> Sum/1
  leaky integration/1(Outport) -> piecewise lin./1

== system TRN_current/Ventrolateral Thalamus/chan5 ==
  BG : Inport  Orientation=down  Port=1  LatchInput=off
  Cortex : Inport  Orientation=down  Port=2  LatchInput=off
  TRN : Inport  Orientation=down  Port=3  LatchInput=off
  TRN1 : Inport  Orientation=down  Port=4  LatchInput=off
  Sum : Sum  Orientation=down  Inputs=++++  SaturateOnIntegerOverflow=on  InputSameDT=on
  leaky integration : Subsystem  Orientation=down
  piecewise lin. : S-Function  Orientation=down  FunctionName=Mpieclin  Parameters=slope,thresh
  weight : Gain  Orientation=down  Gain=W_Ctx  SaturateOnIntegerOverflow=on
  weight1 : Gain  Orientation=down  Gain=W_BG  SaturateOnIntegerOverflow=on
  weight2 : Gain  Orientation=down  Gain=W_TRNwit  SaturateOnIntegerOverflow=on
  weight3 : Gain  Orientation=down  Gain=W_TRNdif  SaturateOnIntegerOverflow=on
  out : Outport  Orientation=down  InitialOutput=0
  wires:
  leaky integration/1(Outport) -> piecewise lin./1
  weight1/1 -> Sum/1
  weight/1 -> Sum/2
  BG/1 -> weight1/1
  Cortex/1 -> weight/1
  weight2/1 -> Sum/3
  TRN/1 -> weight2/1
  TRN1/1 -> weight3/1
  weight3/1 -> Sum/4
  Sum/1 -> leaky integration/1(Inport)
  piecewise lin./1 -> out/1

== system TRN_current/Ventrolateral Thalamus/chan6 ==
  BG : Inport  Orientation=down  Port=1  LatchInput=off
  Cortex : Inport  Orientation=down  Port=2  LatchInput=off
  TRN : Inport  Orientation=down  Port=3  LatchInput=off
  TRN1 : Inport  Orientation=down  Port=4  LatchInput=off
  Sum : Sum  Orientation=down  Inputs=++++  SaturateOnIntegerOverflow=on  InputSameDT=on
  leaky integration : Subsystem  Orientation=down
  piecewise lin. : S-Function  Orientation=down  FunctionName=Mpieclin  Parameters=slope,thresh
  weight : Gain  Orientation=down  Gain=W_Ctx  SaturateOnIntegerOverflow=on
  weight1 : Gain  Orientation=down  Gain=W_BG  SaturateOnIntegerOverflow=on
  weight2 : Gain  Orientation=down  Gain=W_TRNwit  SaturateOnIntegerOverflow=on
  weight3 : Gain  Orientation=down  Gain=W_TRNdif  SaturateOnIntegerOverflow=on
  out : Outport  Orientation=down  InitialOutput=0
  wires:
  piecewise lin./1 -> out/1
  Sum/1 -> leaky integration/1(Inport)
  weight3/1 -> Sum/4
  TRN1/1 -> weight3/1
  TRN/1 -> weight2/1
  weight2/1 -> Sum/3
  Cortex/1 -> weight/1
  BG/1 -> weight1/1
  weight/1 -> Sum/2
  weight1/1 -> Sum/1
  leaky integration/1(Outport) -> piecewise lin./1

== system TRN_current/Basal Ganglia/GPe/2 input channel ==
  Striatum : Inport  Orientation=down  Port=1  LatchInput=off
  STN : Inport  Orientation=down  Port=2  LatchInput=off
  input summation : Subsystem  Orientation=down
  leaky integration : Subsystem  Orientation=down
  piecewise lin. : S-Function  Orientation=down  FunctionName=Mpieclin  Parameters=slope,thresh
  out : Outport  Orientation=down  InitialOutput=0
  wires:
  leaky integration/1(Outport) -> piecewise lin./1
  input summation/1(out_1) -> leaky integration/1(Inport)
  Striatum/1 -> input summation/1(x1)
  STN/1 -> input summation/2(x2)
  piecewise lin./1 -> out/1

== system TRN_current/Basal Ganglia/GPe/2 input channel1 ==
  Striatum : Inport  Orientation=down  Port=1  LatchInput=off
  STN : Inport  Orientation=down  Port=2  LatchInput=off
  input summation : Subsystem  Orientation=down
  leaky integration : Subsystem  Orientation=down
  piecewise lin. : S-Function  Orientation=down  FunctionName=Mpieclin  Parameters=slope,thresh
  out : Outport  Orientation=down  InitialOutput=0
  wires:
  piecewise lin./1 -> out/1
  STN/1 -> input summation/2(x2)
  Striatum/1 -> input summation/1(x1)
  leaky integration/1(Outport) -> piecewise lin./1
  input summation/1(out_1) -> leaky integration/1(Inport)

== system TRN_current/Basal Ganglia/GPe/2 input channel2 ==
  Striatum : Inport  Orientation=down  Port=1  LatchInput=off
  STN : Inport  Orientation=down  Port=2  LatchInput=off
  input summation : Subsystem  Orientation=down
  leaky integration : Subsystem  Orientation=down
  piecewise lin. : S-Function  Orientation=down  FunctionName=Mpieclin  Parameters=slope,thresh
  out : Outport  Orientation=down  InitialOutput=0
  wires:
  input summation/1(out_1) -> leaky integration/1(Inport)
  leaky integration/1(Outport) -> piecewise lin./1
  Striatum/1 -> input summation/1(x1)
  STN/1 -> input summation/2(x2)
  piecewise lin./1 -> out/1

== system TRN_current/Basal Ganglia/GPe/2 input channel3 ==
  Striatum : Inport  Orientation=down  Port=1  LatchInput=off
  STN : Inport  Orientation=down  Port=2  LatchInput=off
  input summation : Subsystem  Orientation=down
  leaky integration : Subsystem  Orientation=down
  piecewise lin. : S-Function  Orientation=down  FunctionName=Mpieclin  Parameters=slope,thresh
  out : Outport  Orientation=down  InitialOutput=0
  wires:
  piecewise lin./1 -> out/1
  STN/1 -> input summation/2(x2)
  Striatum/1 -> input summation/1(x1)
  leaky integration/1(Outport) -> piecewise lin./1
  input summation/1(out_1) -> leaky integration/1(Inport)

== system TRN_current/Basal Ganglia/GPe/2 input channel4 ==
  Striatum : Inport  Orientation=down  Port=1  LatchInput=off
  STN : Inport  Orientation=down  Port=2  LatchInput=off
  input summation : Subsystem  Orientation=down
  leaky integration : Subsystem  Orientation=down
  piecewise lin. : S-Function  Orientation=down  FunctionName=Mpieclin  Parameters=slope,thresh
  out : Outport  Orientation=down  InitialOutput=0
  wires:
  input summation/1(out_1) -> leaky integration/1(Inport)
  leaky integration/1(Outport) -> piecewise lin./1
  Striatum/1 -> input summation/1(x1)
  STN/1 -> input summation/2(x2)
  piecewise lin./1 -> out/1

== system TRN_current/Basal Ganglia/GPe/2 input channel5 ==
  Striatum : Inport  Orientation=down  Port=1  LatchInput=off
  STN : Inport  Orientation=down  Port=2  LatchInput=off
  input summation : Subsystem  Orientation=down
  leaky integration : Subsystem  Orientation=down
  piecewise lin. : S-Function  Orientation=down  FunctionName=Mpieclin  Parameters=slope,thresh
  out : Outport  Orientation=down  InitialOutput=0
  wires:
  piecewise lin./1 -> out/1
  STN/1 -> input summation/2(x2)
  Striatum/1 -> input summation/1(x1)
  leaky integration/1(Outport) -> piecewise lin./1
  input summation/1(out_1) -> leaky integration/1(Inport)

== system TRN_current/Basal Ganglia/GPi/2 input channel ==
  Striatum : Inport  Orientation=down  Port=1  LatchInput=off
  STN : Inport  Orientation=down  Port=2  LatchInput=off
  GPe : Inport  Orientation=down  Port=3  LatchInput=off
  input summation : Subsystem  Orientation=down
  leaky integration : Subsystem  Orientation=down
  piecewise lin. : S-Function  Orientation=down  FunctionName=Mpieclin  Parameters=slope,thresh
  out : Outport  Orientation=down  InitialOutput=0
  wires:
  piecewise lin./1 -> out/1
  STN/1 -> input summation/2(x2)
  Striatum/1 -> input summation/1(x1)
  leaky integration/1(Outport) -> piecewise lin./1
  input summation/1(out_1) -> leaky integration/1(Inport)
  GPe/1 -> input summation/3(x3)

== system TRN_current/Basal Ganglia/GPi/2 input channel1 ==
  Striatum : Inport  Orientation=down  Port=1  LatchInput=off
  STN : Inport  Orientation=down  Port=2  LatchInput=off
  GPe : Inport  Orientation=down  Port=3  LatchInput=off
  input summation : Subsystem  Orientation=down
  leaky integration : Subsystem  Orientation=down
  piecewise lin. : S-Function  Orientation=down  FunctionName=Mpieclin  Parameters=slope,thresh
  out : Outport  Orientation=down  InitialOutput=0
  wires:
  GPe/1 -> input summation/3(x3)
  input summation/1(out_1) -> leaky integration/1(Inport)
  leaky integration/1(Outport) -> piecewise lin./1
  Striatum/1 -> input summation/1(x1)
  STN/1 -> input summation/2(x2)
  piecewise lin./1 -> out/1

== system TRN_current/Basal Ganglia/GPi/2 input channel2 ==
  Striatum : Inport  Orientation=down  Port=1  LatchInput=off
  STN : Inport  Orientation=down  Port=2  LatchInput=off
  GPe : Inport  Orientation=down  Port=3  LatchInput=off
  input summation : Subsystem  Orientation=down
  leaky integration : Subsystem  Orientation=down
  piecewise lin. : S-Function  Orientation=down  FunctionName=Mpieclin  Parameters=slope,thresh
  out : Outport  Orientation=down  InitialOutput=0
  wires:
  piecewise lin./1 -> out/1
  STN/1 -> input summation/2(x2)
  Striatum/1 -> input summation/1(x1)
  leaky integration/1(Outport) -> piecewise lin./1
  input summation/1(out_1) -> leaky integration/1(Inport)
  GPe/1 -> input summation/3(x3)

== system TRN_current/Basal Ganglia/GPi/2 input channel3 ==
  Striatum : Inport  Orientation=down  Port=1  LatchInput=off
  STN : Inport  Orientation=down  Port=2  LatchInput=off
  GPe : Inport  Orientation=down  Port=3  LatchInput=off
  input summation : Subsystem  Orientation=down
  leaky integration : Subsystem  Orientation=down
  piecewise lin. : S-Function  Orientation=down  FunctionName=Mpieclin  Parameters=slope,thresh
  out : Outport  Orientation=down  InitialOutput=0
  wires:
  GPe/1 -> input summation/3(x3)
  input summation/1(out_1) -> leaky integration/1(Inport)
  leaky integration/1(Outport) -> piecewise lin./1
  Striatum/1 -> input summation/1(x1)
  STN/1 -> input summation/2(x2)
  piecewise lin./1 -> out/1

== system TRN_current/Basal Ganglia/GPi/2 input channel4 ==
  Striatum : Inport  Orientation=down  Port=1  LatchInput=off
  STN : Inport  Orientation=down  Port=2  LatchInput=off
  GPe : Inport  Orientation=down  Port=3  LatchInput=off
  input summation : Subsystem  Orientation=down
  leaky integration : Subsystem  Orientation=down
  piecewise lin. : S-Function  Orientation=down  FunctionName=Mpieclin  Parameters=slope,thresh
  out : Outport  Orientation=down  InitialOutput=0
  wires:
  piecewise lin./1 -> out/1
  STN/1 -> input summation/2(x2)
  Striatum/1 -> input summation/1(x1)
  leaky integration/1(Outport) -> piecewise lin./1
  input summation/1(out_1) -> leaky integration/1(Inport)
  GPe/1 -> input summation/3(x3)

== system TRN_current/Basal Ganglia/GPi/2 input channel5 ==
  Striatum : Inport  Orientation=down  Port=1  LatchInput=off
  STN : Inport  Orientation=down  Port=2  LatchInput=off
  GPe : Inport  Orientation=down  Port=3  LatchInput=off
  input summation : Subsystem  Orientation=down
  leaky integration : Subsystem  Orientation=down
  piecewise lin. : S-Function  Orientation=down  FunctionName=Mpieclin  Parameters=slope,thresh
  out : Outport  Orientation=down  InitialOutput=0
  wires:
  GPe/1 -> input summation/3(x3)
  input summation/1(out_1) -> leaky integration/1(Inport)
  leaky integration/1(Outport) -> piecewise lin./1
  Striatum/1 -> input summation/1(x1)
  STN/1 -> input summation/2(x2)
  piecewise lin./1 -> out/1

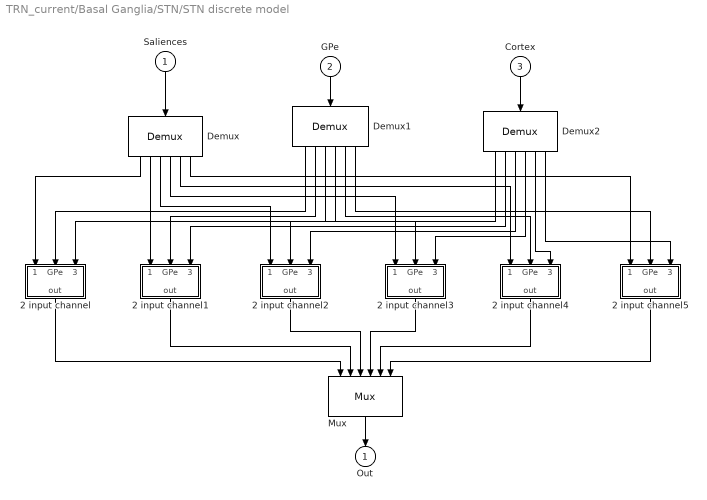
== system TRN_current/Basal Ganglia/STN/STN discrete model ==
  Saliences : Inport  Orientation=down  Port=1  LatchInput=off
  GPe : Inport  Orientation=down  Port=2  LatchInput=off
  Cortex : Inport  Orientation=down  Port=3  LatchInput=off
  2 input channel : Subsystem  Orientation=down
  2 input channel1 : Subsystem  Orientation=down
  2 input channel2 : Subsystem  Orientation=down
  2 input channel3 : Subsystem  Orientation=down
  2 input channel4 : Subsystem  Orientation=down
  2 input channel5 : Subsystem  Orientation=down
  Demux : Demux  Orientation=down  Outputs=6
  Demux1 : Demux  Orientation=down  Outputs=6
  Demux2 : Demux  Orientation=down  Outputs=6
  Mux : Mux  Orientation=down  Inputs=6
  Out : Outport  Orientation=down  InitialOutput=0
  wires:
  Demux/3 -> 2 input channel2/1(Salience)
  Demux/2 -> 2 input channel1/1(Salience)
  Demux/1 -> 2 input channel/1(Salience)
  Saliences/1 -> Demux/1
  Mux/1 -> Out/1
  2 input channel2/1(out) -> Mux/3
  2 input channel1/1(out) -> Mux/2
  2 input channel/1(out) -> Mux/1
  2 input channel3/1(out) -> Mux/4
  2 input channel4/1(out) -> Mux/5
  2 input channel5/1(out) -> Mux/6
  Demux/4 -> 2 input channel3/1(Salience)
  Demux/5 -> 2 input channel4/1(Salience)
  Demux/6 -> 2 input channel5/1(Salience)
  Demux1/1 -> 2 input channel/2(GPe)
  GPe/1 -> Demux1/1
  Demux1/2 -> 2 input channel1/2(GPe)
  Demux1/3 -> 2 input channel2/2(GPe)
  Demux1/4 -> 2 input channel3/2(GPe)
  Demux1/5 -> 2 input channel4/2(GPe)
  Demux1/6 -> 2 input channel5/2(GPe)
  Cortex/1 -> Demux2/1
  Demux2/1 -> 2 input channel/3(Cortex)
  Demux2/2 -> 2 input channel1/3(Cortex)
  Demux2/3 -> 2 input channel2/3(Cortex)
  Demux2/4 -> 2 input channel3/3(Cortex)
  Demux2/5 -> 2 input channel4/3(Cortex)
  Demux2/6 -> 2 input channel5/3(Cortex)
